simulink model "Pendulo_SNL"  (R2014a)
settings: Solver=ode45  StartTime=0.0  StopTime=30  MaxStep=0.01  RelTol=1e-3
values from neighbouring files (symbols this model uses):
  Ci1 = 0    [Data20_Sept_2019 (jose-OptiPlex-7460-AIO_s conflicted copy 2019-10-16).mat]    (also in Masa_Resorte_Duro_Parametros.m; Pendulo_SNL_Parametros.m = 0.785398163397)
  Ci2 = 0    [Data20_Sept_2019 (jose-OptiPlex-7460-AIO_s conflicted copy 2019-10-16).mat]    (also in Masa_Resorte_Duro_Parametros.m; Pendulo_SNL_Parametros.m)
  g = 9.8    [Pendulo_SNL_Parametros.m]
  k = 0.1    [Data20_Sept_2019 (jose-OptiPlex-7460-AIO_s conflicted copy 2019-10-16).mat]    (also in Masa_Resorte_Duro_Parametros.m; Pendulo_SNL_Parametros.m = 0.5)
  L = 0.5    [Pendulo_SNL_Parametros.m]
  m = 1    [Data20_Sept_2019 (jose-OptiPlex-7460-AIO_s conflicted copy 2019-10-16).mat]    (also in Masa_Resorte_Duro_Parametros.m; Pendulo_SNL_Parametros.m)
libraries: simulink x1
settings Model: Creator=Jose  LastModifiedBy=Jose

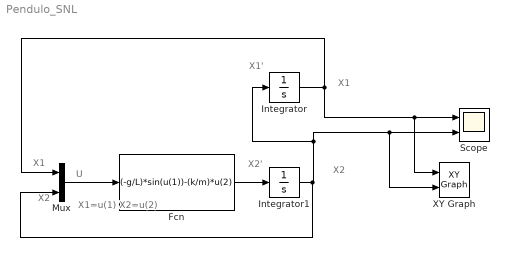
== system Pendulo_SNL ==
  note: X1=u(1)
      | X2=u(2)
  note: U
  note: X2
  note: X1
  note: X2'
  note: X1'
  note: X1
  note: X2
  Fcn : Fcn  Expr=(-g/L)*sin(u(1))-(k/m)*u(2)
  Integrator : Integrator  InitialCondition=Ci1
  Integrator1 : Integrator  InitialCondition=Ci2
  Mux : Mux  Inputs=2
  Scope : Scope  NumInputPorts=2
      settings: YMin=-5~-5  YMax=5~5
  XY Graph : simulink/Sinks/XY Graph  xmin=-1  xmax=3  ymin=-3  ymax=3  st=-1
  wires:
  Integrator1/1 -> Mux/2, XY Graph/2, Scope/2, Integrator/1
  Fcn/1 -> Integrator1/1
  Mux/1 -> Fcn/1
  Integrator/1 -> Mux/1, XY Graph/1, Scope/1
